simulink library "GPIO_Lib"  (Simulink 8.0)
(part 2 of 2)

      mask TypeOptions Pin7_Speed: GPIO_Speed_2MHz | GPIO_Speed_25MHz | GPIO_Speed_50MHz | GPIO_Speed_100MHz
      mask TypeOptions Pin8_Speed: GPIO_Speed_2MHz | GPIO_Speed_25MHz | GPIO_Speed_50MHz | GPIO_Speed_100MHz
      mask TypeOptions Pin9_Speed: GPIO_Speed_2MHz | GPIO_Speed_25MHz | GPIO_Speed_50MHz | GPIO_Speed_100MHz
      mask TypeOptions Pin10_Speed: GPIO_Speed_2MHz | GPIO_Speed_25MHz | GPIO_Speed_50MHz | GPIO_Speed_100MHz
      mask TypeOptions Pin11_Speed: GPIO_Speed_2MHz | GPIO_Speed_25MHz | GPIO_Speed_50MHz | GPIO_Speed_100MHz
      mask TypeOptions Pin12_Speed: GPIO_Speed_2MHz | GPIO_Speed_25MHz | GPIO_Speed_50MHz | GPIO_Speed_100MHz
      mask TypeOptions Pin13_Speed: GPIO_Speed_2MHz | GPIO_Speed_25MHz | GPIO_Speed_50MHz | GPIO_Speed_100MHz
      mask TypeOptions Pin14_Speed: GPIO_Speed_2MHz | GPIO_Speed_25MHz | GPIO_Speed_50MHz | GPIO_Speed_100MHz
      mask TypeOptions Pin15_Speed: GPIO_Speed_2MHz | GPIO_Speed_25MHz | GPIO_Speed_50MHz | GPIO_Speed_100MHz
      mask TypeOptions Pin0_Mode: GPIO_Mode_IN | GPIO_Mode_OUT | GPIO_Mode_AF | GPIO_Mode_AN
      mask Callback Pin0_Mode: GPIOG_Config_callback('mode0');
      mask TypeOptions Pin1_Mode: GPIO_Mode_IN | GPIO_Mode_OUT | GPIO_Mode_AF | GPIO_Mode_AN
      mask Callback Pin1_Mode: GPIOG_Config_callback('mode1');
      mask TypeOptions Pin2_Mode: GPIO_Mode_IN | GPIO_Mode_OUT | GPIO_Mode_AF | GPIO_Mode_AN
      mask Callback Pin2_Mode: GPIOG_Config_callback('mode2');
      mask TypeOptions Pin3_Mode: GPIO_Mode_IN | GPIO_Mode_OUT | GPIO_Mode_AF | GPIO_Mode_AN
      mask Callback Pin3_Mode: GPIOG_Config_callback('mode3');
      mask TypeOptions Pin4_Mode: GPIO_Mode_IN | GPIO_Mode_OUT | GPIO_Mode_AF | GPIO_Mode_AN
      mask Callback Pin4_Mode: GPIOA_Config_callback('mode4');
      mask TypeOptions Pin5_Mode: GPIO_Mode_IN | GPIO_Mode_OUT | GPIO_Mode_AF | GPIO_Mode_AN
      mask Callback Pin5_Mode: GPIOG_Config_callback('mode5');
      mask TypeOptions Pin6_Mode: GPIO_Mode_IN | GPIO_Mode_OUT | GPIO_Mode_AF | GPIO_Mode_AN
      mask Callback Pin6_Mode: GPIOG_Config_callback('mode6');
      mask TypeOptions Pin7_Mode: GPIO_Mode_IN | GPIO_Mode_OUT | GPIO_Mode_AF | GPIO_Mode_AN
      mask Callback Pin7_Mode: GPIOG_Config_callback('mode7');
      mask TypeOptions Pin8_Mode: GPIO_Mode_IN | GPIO_Mode_OUT | GPIO_Mode_AF | GPIO_Mode_AN
      mask Callback Pin8_Mode: GPIOG_Config_callback('mode8');
      mask TypeOptions Pin9_Mode: GPIO_Mode_IN | GPIO_Mode_OUT | GPIO_Mode_AF | GPIO_Mode_AN
      mask Callback Pin9_Mode: GPIOG_Config_callback('mode9');
      mask TypeOptions Pin10_Mode: GPIO_Mode_IN | GPIO_Mode_OUT | GPIO_Mode_AF | GPIO_Mode_AN
      mask Callback Pin10_Mode: GPIOG_Config_callback('mode10');
      mask TypeOptions Pin11_Mode: GPIO_Mode_IN | GPIO_Mode_OUT | GPIO_Mode_AF | GPIO_Mode_AN
      mask Callback Pin11_Mode: GPIOG_Config_callback('mode11');
      mask TypeOptions Pin12_Mode: GPIO_Mode_IN | GPIO_Mode_OUT | GPIO_Mode_AF | GPIO_Mode_AN
      mask Callback Pin12_Mode: GPIOG_Config_callback('mode12');
      mask TypeOptions Pin13_Mode: GPIO_Mode_IN | GPIO_Mode_OUT | GPIO_Mode_AF | GPIO_Mode_AN
      mask Callback Pin13_Mode: GPIOG_Config_callback('mode13');
      mask TypeOptions Pin14_Mode: GPIO_Mode_IN | GPIO_Mode_OUT | GPIO_Mode_AF | GPIO_Mode_AN
      mask Callback Pin14_Mode: GPIOG_Config_callback('mode14');
      mask TypeOptions Pin15_Mode: GPIO_Mode_IN | GPIO_Mode_OUT | GPIO_Mode_AF | GPIO_Mode_AN
      mask Callback Pin15_Mode: GPIOG_Config_callback('mode15');
      mask TypeOptions Pin0_Type: GPIO_OType_PP | GPIO_OType_OD
      mask TypeOptions Pin1_Type: GPIO_OType_PP | GPIO_OType_OD
      mask TypeOptions Pin2_Type: GPIO_OType_PP | GPIO_OType_OD
      mask TypeOptions Pin3_Type: GPIO_OType_PP | GPIO_OType_OD
      mask TypeOptions Pin4_Type: GPIO_OType_PP | GPIO_OType_OD
      mask TypeOptions Pin5_Type: GPIO_OType_PP | GPIO_OType_OD
      mask TypeOptions Pin6_Type: GPIO_OType_PP | GPIO_OType_OD
      mask TypeOptions Pin7_Type: GPIO_OType_PP | GPIO_OType_OD
      mask TypeOptions Pin8_Type: GPIO_OType_PP | GPIO_OType_OD
      mask TypeOptions Pin9_Type: GPIO_OType_PP | GPIO_OType_OD
      mask TypeOptions Pin10_Type: GPIO_OType_PP | GPIO_OType_OD
      mask TypeOptions Pin11_Type: GPIO_OType_PP | GPIO_OType_OD
      mask TypeOptions Pin12_Type: GPIO_OType_PP | GPIO_OType_OD
      mask TypeOptions Pin13_Type: GPIO_OType_PP | GPIO_OType_OD
      mask TypeOptions Pin14_Type: GPIO_OType_PP | GPIO_OType_OD
      mask TypeOptions Pin15_Type: GPIO_OType_PP | GPIO_OType_OD
      mask TypeOptions Pin0_PuPd: GPIO_PuPd_NOPULL | GPIO_PuPd_UP | GPIO_PuPd_DOWN
      mask TypeOptions Pin1_PuPd: GPIO_PuPd_NOPULL | GPIO_PuPd_UP | GPIO_PuPd_DOWN
      mask TypeOptions Pin2_PuPd: GPIO_PuPd_NOPULL | GPIO_PuPd_UP | GPIO_PuPd_DOWN
      mask TypeOptions Pin3_PuPd: GPIO_PuPd_NOPULL | GPIO_PuPd_UP | GPIO_PuPd_DOWN
      mask TypeOptions Pin4_PuPd: GPIO_PuPd_NOPULL | GPIO_PuPd_UP | GPIO_PuPd_DOWN
      mask TypeOptions Pin5_PuPd: GPIO_PuPd_NOPULL | GPIO_PuPd_UP | GPIO_PuPd_DOWN
      mask TypeOptions Pin6_PuPd: GPIO_PuPd_NOPULL | GPIO_PuPd_UP | GPIO_PuPd_DOWN
      mask TypeOptions Pin7_PuPd: GPIO_PuPd_NOPULL | GPIO_PuPd_UP | GPIO_PuPd_DOWN
      mask TypeOptions Pin8_PuPd: GPIO_PuPd_NOPULL | GPIO_PuPd_UP | GPIO_PuPd_DOWN
      mask TypeOptions Pin9_PuPd: GPIO_PuPd_NOPULL | GPIO_PuPd_UP | GPIO_PuPd_DOWN
      mask TypeOptions Pin10_PuPd: GPIO_PuPd_NOPULL | GPIO_PuPd_UP | GPIO_PuPd_DOWN
      mask TypeOptions Pin11_PuPd: GPIO_PuPd_NOPULL | GPIO_PuPd_UP | GPIO_PuPd_DOWN
      mask TypeOptions Pin12_PuPd: GPIO_PuPd_NOPULL | GPIO_PuPd_UP | GPIO_PuPd_DOWN
      mask TypeOptions Pin13_PuPd: GPIO_PuPd_NOPULL | GPIO_PuPd_UP | GPIO_PuPd_DOWN
      mask TypeOptions Pin14_PuPd: GPIO_PuPd_NOPULL | GPIO_PuPd_UP | GPIO_PuPd_DOWN
      mask TypeOptions Pin15_PuPd: GPIO_PuPd_NOPULL | GPIO_PuPd_UP | GPIO_PuPd_DOWN
      mask TypeOptions Pin0_AF: GPIO_AF_FSMC | GPIO_AF_EVENTOUT
      mask TypeOptions Pin1_AF: GPIO_AF_FSMC | GPIO_AF_EVENTOUT
      mask TypeOptions Pin2_AF: GPIO_AF_FSMC | GPIO_AF_EVENTOUT
      mask TypeOptions Pin3_AF: GPIO_AF_FSMC | GPIO_AF_EVENTOUT
      mask TypeOptions Pin4_AF: GPIO_AF_FSMC | GPIO_AF_EVENTOUT
      mask TypeOptions Pin5_AF: GPIO_AF_FSMC | GPIO_AF_EVENTOUT
      mask TypeOptions Pin6_AF: GPIO_AF_FSMC | GPIO_AF_EVENTOUT
      mask TypeOptions Pin7_AF: GPIO_AF_USART6 | GPIO_AF_FSMC | GPIO_AF_EVENTOUT
      mask TypeOptions Pin8_AF: GPIO_AF_USART6 | GPIO_AF_ETH | GPIO_AF_EVENTOUT
      mask TypeOptions Pin9_AF: GPIO_AF_USART6 | GPIO_AF_FSMC | GPIO_AF_EVENTOUT
      mask TypeOptions Pin10_AF: GPIO_AF_FSMC | GPIO_AF_EVENTOUT
      mask TypeOptions Pin11_AF: GPIO_AF_ETH | GPIO_AF_FSMC | GPIO_AF_EVENTOUT
      mask TypeOptions Pin12_AF: GPIO_AF_USART6 | GPIO_AF_FSMC | GPIO_AF_EVENTOUT
      mask TypeOptions Pin13_AF: GPIO_AF_USART6 | GPIO_AF_ETH | GPIO_AF_FSMC | GPIO_AF_EVENTOUT
      mask TypeOptions Pin14_AF: GPIO_AF_USART6 | GPIO_AF_ETH | GPIO_AF_FSMC | GPIO_AF_EVENTOUT
      mask TypeOptions Pin15_AF: GPIO_AF_USART6 | GPIO_AF_DCMI | GPIO_AF_EVENTOUT
      mask Display:
      | color('blue'); text(0.6, 0.90, 'STM32F4xx', 'horizontalalignment', 'right');color('black'); text(0.50, 0.12, 'GPIOG_Config', 'horizontalAlignment','center');
      | image(imread('ST.bmp','bmp'),'top-right');
  GPIOH_Config : S-Function  LoadFcn=|  FunctionName=GPIOH_Config  Parameters=Pin0_Use,Pin1_Use,Pin2_Use,Pin3_Use,Pin4_Use,Pin5_Use,Pin6_Use,Pin7_Use,Pin8_Use,Pin9_Use,Pin10_Use,Pin11_Use,Pin12_Use,Pin13_Use,Pin14_Use,Pin15_Use,Pin0_Speed,Pin1_Speed,Pin2_Speed,Pin3_Speed,Pin4_Speed,Pin5_Speed,Pin6_Speed,Pin7_Speed,Pin8_Speed,Pin9_Speed,Pin10_Speed,Pin11_Speed,Pin12_Speed,Pin13_Speed,Pin14_Speed,Pin15_Speed,Pin0_Mode,Pin1_Mode,Pin2_Mode,Pin3_Mode,Pin4_Mode,Pin5_Mode,Pin6_Mode,Pin7_Mode,Pin8_Mode,Pin9_Mode,Pin10_Mode,Pin11_Mode,Pin12_Mode,Pin13_Mode,Pin14_Mode,Pin15_Mode,Pin0_Type,Pin1_Type,Pin2_Type,Pin3_Type,Pin4_Type,Pin5_Type,Pin6_Type,Pin7_Type,Pin8_Type,Pin9_Type,Pin10_Type,Pin11_Type,Pin12_Type,Pin13_Type,Pin14_Type,Pin15_Type,Pin0_PuPd,Pin1_PuPd,Pin2_PuPd,Pin3_PuPd,Pin4_PuPd,Pin5_PuPd,Pin6_PuPd,Pin7_PuPd,Pin8_PuPd,Pin9_PuPd,Pin10_PuPd,Pin11_PuPd,Pin12_PuPd,Pin13_PuPd,Pin14_PuPd,Pin15_PuPd,Pin2_AF,Pin3_AF,Pin4_AF,Pin5_AF,Pin6_AF,Pin7_AF,Pin8_AF,Pin9_AF,Pin10_AF,Pin11_AF,Pin12_AF,Pin13_AF,Pin14_AF,Pin15_AF,Pin0_Set,Pin1_Set,Pin2_Set,Pin3_Set,Pin4_Set,Pin5_Set,Pin6_Set,Pin7_Set,Pin8_Set,Pin9_Set,Pin10_Set,Pin11_Set,Pin12_Set,Pin13_Set,Pin14_Set,Pin15_Set  EnableBusSupport=off  mask(GPIOH_Config){Pin0_Use=off, Pin1_Use=off, Pin2_Use=off, Pin3_Use=off, Pin4_Use=off, Pin5_Use=off, Pin6_Use=off, Pin7_Use=off, Pin8_Use=off, Pin9_Use=off, Pin10_Use=off, Pin11_Use=off, Pin12_Use=off, Pin13_Use=off, Pin14_Use=off, Pin15_Use=off, Pin0_Speed=GPIO_Speed_2MHz, Pin1_Speed=GPIO_Speed_2MHz, Pin2_Speed=GPIO_Speed_2MHz, Pin3_Speed=GPIO_Speed_2MHz, Pin4_Speed=GPIO_Speed_2MHz, Pin5_Speed=GPIO_Speed_2MHz, Pin6_Speed=GPIO_Speed_2MHz, Pin7_Speed=GPIO_Speed_2MHz, Pin8_Speed=GPIO_Speed_2MHz, Pin9_Speed=GPIO_Speed_2MHz, Pin10_Speed=GPIO_Speed_2MHz, Pin11_Speed=GPIO_Speed_2MHz, Pin12_Speed=GPIO_Speed_2MHz, Pin13_Speed=GPIO_Speed_2MHz, Pin14_Speed=GPIO_Speed_2MHz, Pin15_Speed=GPIO_Speed_2MHz, Pin0_Mode=GPIO_Mode_OUT, Pin1_Mode=GPIO_Mode_OUT, Pin2_Mode=GPIO_Mode_OUT, Pin3_Mode=GPIO_Mode_OUT, Pin4_Mode=GPIO_Mode_OUT, Pin5_Mode=GPIO_Mode_OUT, Pin6_Mode=GPIO_Mode_OUT, Pin7_Mode=GPIO_Mode_OUT, Pin8_Mode=GPIO_Mode_OUT, Pin9_Mode=GPIO_Mode_OUT, Pin10_Mode=GPIO_Mode_OUT, Pin11_Mode=GPIO_Mode_OUT, Pin12_Mode=GPIO_Mode_OUT, Pin13_Mode=GPIO_Mode_OUT, Pin14_Mode=GPIO_Mode_OUT, Pin15_Mode=GPIO_Mode_OUT, Pin0_Type=GPIO_OType_PP, Pin1_Type=GPIO_OType_PP, Pin2_Type=GPIO_OType_PP, Pin3_Type=GPIO_OType_PP, Pin4_Type=GPIO_OType_PP, Pin5_Type=GPIO_OType_PP, Pin6_Type=GPIO_OType_PP, Pin7_Type=GPIO_OType_PP, Pin8_Type=GPIO_OType_PP, Pin9_Type=GPIO_OType_PP, Pin10_Type=GPIO_OType_PP, Pin11_Type=GPIO_OType_PP, Pin12_Type=GPIO_OType_PP, Pin13_Type=GPIO_OType_PP, Pin14_Type=GPIO_OType_PP, Pin15_Type=GPIO_OType_PP, Pin0_PuPd=GPIO_PuPd_NOPULL, Pin1_PuPd=GPIO_PuPd_NOPULL, Pin2_PuPd=GPIO_PuPd_NOPULL, Pin3_PuPd=GPIO_PuPd_NOPULL, Pin4_PuPd=GPIO_PuPd_NOPULL, Pin5_PuPd=GPIO_PuPd_NOPULL, Pin6_PuPd=GPIO_PuPd_NOPULL, Pin7_PuPd=GPIO_PuPd_NOPULL, Pin8_PuPd=GPIO_PuPd_NOPULL, Pin9_PuPd=GPIO_PuPd_NOPULL, Pin10_PuPd=GPIO_PuPd_NOPULL, Pin11_PuPd=GPIO_PuPd_NOPULL, Pin12_PuPd=GPIO_PuPd_NOPULL, Pin13_PuPd=GPIO_PuPd_NOPULL, Pin14_PuPd=GPIO_PuPd_NOPULL, Pin15_PuPd=GPIO_PuPd_NOPULL, Pin2_AF=GPIO_AF_ETH, Pin3_AF=GPIO_AF_ETH, Pin4_AF=GPIO_AF_I2C2, Pin5_AF=GPIO_AF_EVENTOUT, Pin6_AF=GPIO_AF_I2C2, Pin7_AF=GPIO_AF_I2C3, Pin8_AF=GPIO_AF_I2C3, Pin9_AF=GPIO_AF_I2C3, Pin10_AF=GPIO_AF_TIM5, Pin11_AF=GPIO_AF_TIM5, Pin12_AF=GPIO_AF_TIM5, Pin13_AF=GPIO_AF_TIM8, Pin14_AF=GPIO_AF_TIM8, Pin15_AF=GPIO_AF_EVENTOUT, Pin0_Set=off, Pin1_Set=off, Pin2_Set=off, Pin3_Set=off, Pin4_Set=off, Pin5_Set=off, Pin6_Set=off, Pin7_Set=off, Pin8_Set=off, Pin9_Set=off, Pin10_Set=off, Pin11_Set=off, Pin12_Set=off, Pin13_Set=off, Pin14_Set=off, Pin15_Set=off}
      | libFiles =    updatePrefs('get','stm32f4listLibFiles');          libFiles2Build = updatePrefs('get','stm32f4listLibBuildFiles');
      |                                                                                                                                 
      | gpio = strcmp('stm32f4xx_gpio.c',{libFiles(:).name});                                                                           
      | libFiles2Build(gpio) = libFiles2Build(gpio) + 1;                                                                                
      | rcc = strcmp('stm32f4xx_rcc.c',{libFiles(:).name}) ;                                                                            
      | libFiles2Build(rcc) = libFiles2Build(rcc) + 1;                                                                                  
      |                                                                                                                                 
      | updatePrefs('set','stm32f4listLibBuildFiles',libFiles2Build);                                                                   
      | clear gpio rcc  libFiles                                                                                                        
      | clear libFiles2Build
      mask prompts: Pin0_Use "Pin used"; Pin1_Use "Pin used"; Pin2_Use "Pin used"; Pin3_Use "Pin used"; Pin4_Use "Pin used"; Pin5_Use "Pin used"; Pin6_Use "Pin used"; Pin7_Use "Pin used"; Pin8_Use "Pin used"; Pin9_Use "Pin used"; Pin10_Use "Pin used"; Pin11_Use "Pin used"; Pin12_Use "Pin used"; Pin13_Use "Pin used"; Pin14_Use "Pin used"; Pin15_Use "Pin used"; Pin0_Speed "Maximum frequency"; Pin1_Speed "Maximum frequency"; Pin2_Speed "Maximum frequency"; Pin3_Speed "Maximum frequency"; Pin4_Speed "Maximum frequency"; Pin5_Speed "Maximum frequency"; Pin6_Speed "Maximum frequency"; Pin7_Speed "Maximum frequency"; Pin8_Speed "Maximum frequency"; Pin9_Speed "Maximum frequency"; Pin10_Speed "Maximum frequency"; Pin11_Speed "Maximum frequency"; Pin12_Speed "Maximum frequency"; Pin13_Speed "Maximum frequency"; Pin14_Speed "Maximum frequency"; Pin15_Speed "Maximum frequency"; Pin0_Mode "Configuration mode"; Pin1_Mode "Configuration mode"; Pin2_Mode "Configuration mode"; Pin3_Mode "Configuration mode"; Pin4_Mode "Configuration mode"; Pin5_Mode "Configuration mode"; Pin6_Mode "Configuration mode"; Pin7_Mode "Configuration mode"; Pin8_Mode "Configuration mode"; Pin9_Mode "Configuration mode"; Pin10_Mode "Configuration mode"; Pin11_Mode "Configuration mode"; Pin12_Mode "Configuration mode"; Pin13_Mode "Configuration mode"; Pin14_Mode "Configuration mode"; Pin15_Mode "Configuration mode"; Pin0_Type "Configuration output type"; Pin1_Type "Configuration output type"; Pin2_Type "Configuration output type"; Pin3_Type "Configuration output type"; Pin4_Type "Configuration output type"; Pin5_Type "Configuration output type"; Pin6_Type "Configuration output type"; Pin7_Type "Configuration output type"; Pin8_Type "Configuration output type"; Pin9_Type "Configuration output type"; Pin10_Type "Configuration output type"; Pin11_Type "Configuration output type"; Pin12_Type "Configuration output type"; Pin13_Type "Configuration output type"; Pin14_Type "Configuration output type"; Pin15_Type "Configuration output type"; Pin0_PuPd "Configuration PullUp PullDown"; Pin1_PuPd "Configuration PullUp PullDown"; Pin2_PuPd "Configuration PullUp PullDown"; Pin3_PuPd "Configuration PullUp PullDown"; Pin4_PuPd "Configuration PullUp PullDown"; Pin5_PuPd "Configuration PullUp PullDown"; Pin6_PuPd "Configuration PullUp PullDown"; Pin7_PuPd "Configuration PullUp PullDown"; Pin8_PuPd "Configuration PullUp PullDown"; Pin9_PuPd "Configuration PullUp PullDown"; Pin10_PuPd "Configuration PullUp PullDown"; Pin11_PuPd "Configuration PullUp PullDown"; Pin12_PuPd "Configuration PullUp PullDown"; Pin13_PuPd "Configuration PullUp PullDown"; Pin14_PuPd "Configuration PullUp PullDown"; Pin15_PuPd "Configuration PullUp PullDown"; Pin2_AF "Alternate Function"; Pin3_AF "Alternate Function"; Pin4_AF "Alternate Function"; Pin5_AF "Alternate Function"; Pin6_AF "Alternate Function"; Pin7_AF "Alternate Function"; Pin8_AF "Alternate Function"; Pin9_AF "Alternate Function"; Pin10_AF "Alternate Function"; Pin11_AF "Alternate Function"; Pin12_AF "Alternate Function"; Pin13_AF "Alternate Function"; Pin14_AF "Alternate Function"; Pin15_AF "Alternate Function"; Pin0_Set "Set High initial value"; Pin1_Set "Set High initial value"; Pin2_Set "Set High initial value"; Pin3_Set "Set High initial value"; Pin4_Set "Set High initial value"; Pin5_Set "Set High initial value"; Pin6_Set "Set High initial value"; Pin7_Set "Set High initial value"; Pin8_Set "Set High initial value"; Pin9_Set "Set High initial value"; Pin10_Set "Set High initial value"; Pin11_Set "Set High initial value"; Pin12_Set "Set High initial value"; Pin13_Set "Set High initial value"; Pin14_Set "Set High initial value"; Pin15_Set "Set High initial value"
      mask help:
      | GPIO (General Purpose In/Out) PortH configuration:
      | Configure PortH, Pin0 to Pin15 as input, output, Analogic or Alternate function.
      | Maximum GPIO speed is 2Mhz, 25Mhz, 50Mhz or 100Mhz.
      | Output is PushPull or OpenDrain.
      | Input is PullUp, PullDown, PullUpPullDown or No pull.
      | Alternate function is different for each pin. (No AF for Pin0 and Pin1)
      settings: CopyFcn=|
      | pathTmf = updatePrefs('get','stm32f4RootPath');
      | if isempty(pathTmf)
      | h = errordlg('Add STM32F4xx repository to Matlab default path or set System target file to stm32F4xx.tlc before!' ,'STM32F4xx','modal');
      | close(h);
      | clear h
      | end
      | libFiles =    updatePrefs('get','stm32f4listLibFiles');          libFiles2Build = updatePrefs('get','stm32f4listLibBuildFiles');
      | gpio = strcmp('stm32f4xx_gpio.c',{libFiles(:).name});
      | libFiles2Build(gpio) = libFiles2Build(gpio) + 1;
      | rcc = strcmp('stm32f4xx_rcc.c',{libFiles(:).name}) ;
      | libFiles2Build(rcc) = libFiles2Build(rcc) + 1;
      | updatePrefs('set','stm32f4listLibBuildFiles',libFiles2Build);
      | clear gpio rcc  pathTmf libFiles
      | clear libFiles2Build
      settings: DeleteFcn=|
      | libFiles =    updatePrefs('get','stm32f4listLibFiles');          libFiles2Build = updatePrefs('get','stm32f4listLibBuildFiles');
      | gpio = strcmp('stm32f4xx_gpio.c',{libFiles(:).name});
      | libFiles2Build(gpio) = libFiles2Build(gpio) - 1;  if(libFiles2Build(gpio) <0)
      | libFiles2Build(gpio)  = 0;                                  end
      | rcc = strcmp('stm32f4xx_rcc.c',{libFiles(:).name}) ;
      | libFiles2Build(rcc) = libFiles2Build(rcc) - 1;    if(libFiles2Build(rcc) <0)
      | libFiles2Build(rcc)  = 0;                                  end
      | updatePrefs('set','stm32f4listLibBuildFiles',libFiles2Build);
      | clear gpio rcc  libFiles  libFiles2Build
      settings: UndoDeleteFcn=|
      | libFiles =    updatePrefs('get','stm32f4listLibFiles');          libFiles2Build = updatePrefs('get','stm32f4listLibBuildFiles');
      | gpio = strcmp('stm32f4xx_gpio.c',{libFiles(:).name});
      | libFiles2Build(gpio) = libFiles2Build(gpio) + 1;
      | rcc = strcmp('stm32f4xx_rcc.c',{libFiles(:).name}) ;
      | libFiles2Build(rcc) = libFiles2Build(rcc) + 1;
      | updatePrefs('set','stm32f4listLibBuildFiles',libFiles2Build);
      | clear gpio rcc  libFiles
      | clear libFiles2Build
      mask Help: web('help_GPIOH_Config.html', '-helpbrowser')
      mask Callback Pin0_Use: GPIOH_Config_callback('use0');
      mask Callback Pin1_Use: GPIOH_Config_callback('use1');
      mask Callback Pin2_Use: GPIOH_Config_callback('use2');
      mask Callback Pin3_Use: GPIOH_Config_callback('use3');
      mask Callback Pin4_Use: GPIOH_Config_callback('use4');
      mask Callback Pin5_Use: GPIOH_Config_callback('use5');
      mask Callback Pin6_Use: GPIOH_Config_callback('use6');
      mask Callback Pin7_Use: GPIOH_Config_callback('use7');
      mask Callback Pin8_Use: GPIOH_Config_callback('use8');
      mask Callback Pin9_Use: GPIOH_Config_callback('use9');
      mask Callback Pin10_Use: GPIOA_Config_callback('use10');
      mask Callback Pin11_Use: GPIOH_Config_callback('use11');
      mask Callback Pin12_Use: GPIOH_Config_callback('use12');
      mask Callback Pin13_Use: GPIOH_Config_callback('use13');
      mask Callback Pin14_Use: GPIOH_Config_callback('use14');
      mask Callback Pin15_Use: GPIOH_Config_callback('use15');
      mask TypeOptions Pin0_Speed: GPIO_Speed_2MHz | GPIO_Speed_25MHz | GPIO_Speed_50MHz | GPIO_Speed_100MHz
      mask TypeOptions Pin1_Speed: GPIO_Speed_2MHz | GPIO_Speed_25MHz | GPIO_Speed_50MHz | GPIO_Speed_100MHz
      mask TypeOptions Pin2_Speed: GPIO_Speed_2MHz | GPIO_Speed_25MHz | GPIO_Speed_50MHz | GPIO_Speed_100MHz
      mask TypeOptions Pin3_Speed: GPIO_Speed_2MHz | GPIO_Speed_25MHz | GPIO_Speed_50MHz | GPIO_Speed_100MHz
      mask TypeOptions Pin4_Speed: GPIO_Speed_2MHz | GPIO_Speed_25MHz | GPIO_Speed_50MHz | GPIO_Speed_100MHz
      mask TypeOptions Pin5_Speed: GPIO_Speed_2MHz | GPIO_Speed_25MHz | GPIO_Speed_50MHz | GPIO_Speed_100MHz
      mask TypeOptions Pin6_Speed: GPIO_Speed_2MHz | GPIO_Speed_25MHz | GPIO_Speed_50MHz | GPIO_Speed_100MHz
      mask TypeOptions Pin7_Speed: GPIO_Speed_2MHz | GPIO_Speed_25MHz | GPIO_Speed_50MHz | GPIO_Speed_100MHz
      mask TypeOptions Pin8_Speed: GPIO_Speed_2MHz | GPIO_Speed_25MHz | GPIO_Speed_50MHz | GPIO_Speed_100MHz
      mask TypeOptions Pin9_Speed: GPIO_Speed_2MHz | GPIO_Speed_25MHz | GPIO_Speed_50MHz | GPIO_Speed_100MHz
      mask TypeOptions Pin10_Speed: GPIO_Speed_2MHz | GPIO_Speed_25MHz | GPIO_Speed_50MHz | GPIO_Speed_100MHz
      mask TypeOptions Pin11_Speed: GPIO_Speed_2MHz | GPIO_Speed_25MHz | GPIO_Speed_50MHz | GPIO_Speed_100MHz
      mask TypeOptions Pin12_Speed: GPIO_Speed_2MHz | GPIO_Speed_25MHz | GPIO_Speed_50MHz | GPIO_Speed_100MHz
      mask TypeOptions Pin13_Speed: GPIO_Speed_2MHz | GPIO_Speed_25MHz | GPIO_Speed_50MHz | GPIO_Speed_100MHz
      mask TypeOptions Pin14_Speed: GPIO_Speed_2MHz | GPIO_Speed_25MHz | GPIO_Speed_50MHz | GPIO_Speed_100MHz
      mask TypeOptions Pin15_Speed: GPIO_Speed_2MHz | GPIO_Speed_25MHz | GPIO_Speed_50MHz | GPIO_Speed_100MHz
      mask TypeOptions Pin0_Mode: GPIO_Mode_IN | GPIO_Mode_OUT | GPIO_Mode_AN
      mask Callback Pin0_Mode: GPIOH_Config_callback('mode0');
      mask TypeOptions Pin1_Mode: GPIO_Mode_IN | GPIO_Mode_OUT | GPIO_Mode_AN
      mask Callback Pin1_Mode: GPIOH_Config_callback('mode1');
      mask TypeOptions Pin2_Mode: GPIO_Mode_IN | GPIO_Mode_OUT | GPIO_Mode_AF | GPIO_Mode_AN
      mask Callback Pin2_Mode: GPIOH_Config_callback('mode2');
      mask TypeOptions Pin3_Mode: GPIO_Mode_IN | GPIO_Mode_OUT | GPIO_Mode_AF | GPIO_Mode_AN
      mask Callback Pin3_Mode: GPIOH_Config_callback('mode3');
      mask TypeOptions Pin4_Mode: GPIO_Mode_IN | GPIO_Mode_OUT | GPIO_Mode_AF | GPIO_Mode_AN
      mask Callback Pin4_Mode: GPIOA_Config_callback('mode4');
      mask TypeOptions Pin5_Mode: GPIO_Mode_IN | GPIO_Mode_OUT | GPIO_Mode_AF | GPIO_Mode_AN
      mask Callback Pin5_Mode: GPIOH_Config_callback('mode5');
      mask TypeOptions Pin6_Mode: GPIO_Mode_IN | GPIO_Mode_OUT | GPIO_Mode_AF | GPIO_Mode_AN
      mask Callback Pin6_Mode: GPIOH_Config_callback('mode6');
      mask TypeOptions Pin7_Mode: GPIO_Mode_IN | GPIO_Mode_OUT | GPIO_Mode_AF | GPIO_Mode_AN
      mask Callback Pin7_Mode: GPIOH_Config_callback('mode7');
      mask TypeOptions Pin8_Mode: GPIO_Mode_IN | GPIO_Mode_OUT | GPIO_Mode_AF | GPIO_Mode_AN
      mask Callback Pin8_Mode: GPIOH_Config_callback('mode8');
      mask TypeOptions Pin9_Mode: GPIO_Mode_IN | GPIO_Mode_OUT | GPIO_Mode_AF | GPIO_Mode_AN
      mask Callback Pin9_Mode: GPIOH_Config_callback('mode9');
      mask TypeOptions Pin10_Mode: GPIO_Mode_IN | GPIO_Mode_OUT | GPIO_Mode_AF | GPIO_Mode_AN
      mask Callback Pin10_Mode: GPIOH_Config_callback('mode10');
      mask TypeOptions Pin11_Mode: GPIO_Mode_IN | GPIO_Mode_OUT | GPIO_Mode_AF | GPIO_Mode_AN
      mask Callback Pin11_Mode: GPIOH_Config_callback('mode11');
      mask TypeOptions Pin12_Mode: GPIO_Mode_IN | GPIO_Mode_OUT | GPIO_Mode_AF | GPIO_Mode_AN
      mask Callback Pin12_Mode: GPIOH_Config_callback('mode12');
      mask TypeOptions Pin13_Mode: GPIO_Mode_IN | GPIO_Mode_OUT | GPIO_Mode_AF | GPIO_Mode_AN
      mask Callback Pin13_Mode: GPIOH_Config_callback('mode13');
      mask TypeOptions Pin14_Mode: GPIO_Mode_IN | GPIO_Mode_OUT | GPIO_Mode_AF | GPIO_Mode_AN
      mask Callback Pin14_Mode: GPIOH_Config_callback('mode14');
      mask TypeOptions Pin15_Mode: GPIO_Mode_IN | GPIO_Mode_OUT | GPIO_Mode_AF | GPIO_Mode_AN
      mask Callback Pin15_Mode: GPIOH_Config_callback('mode15');
      mask TypeOptions Pin0_Type: GPIO_OType_PP | GPIO_OType_OD
      mask TypeOptions Pin1_Type: GPIO_OType_PP | GPIO_OType_OD
      mask TypeOptions Pin2_Type: GPIO_OType_PP | GPIO_OType_OD
      mask TypeOptions Pin3_Type: GPIO_OType_PP | GPIO_OType_OD
      mask TypeOptions Pin4_Type: GPIO_OType_PP | GPIO_OType_OD
      mask TypeOptions Pin5_Type: GPIO_OType_PP | GPIO_OType_OD
      mask TypeOptions Pin6_Type: GPIO_OType_PP | GPIO_OType_OD
      mask TypeOptions Pin7_Type: GPIO_OType_PP | GPIO_OType_OD
      mask TypeOptions Pin8_Type: GPIO_OType_PP | GPIO_OType_OD
      mask TypeOptions Pin9_Type: GPIO_OType_PP | GPIO_OType_OD
      mask TypeOptions Pin10_Type: GPIO_OType_PP | GPIO_OType_OD
      mask TypeOptions Pin11_Type: GPIO_OType_PP | GPIO_OType_OD
      mask TypeOptions Pin12_Type: GPIO_OType_PP | GPIO_OType_OD
      mask TypeOptions Pin13_Type: GPIO_OType_PP | GPIO_OType_OD
      mask TypeOptions Pin14_Type: GPIO_OType_PP | GPIO_OType_OD
      mask TypeOptions Pin15_Type: GPIO_OType_PP | GPIO_OType_OD
      mask TypeOptions Pin0_PuPd: GPIO_PuPd_NOPULL | GPIO_PuPd_UP | GPIO_PuPd_DOWN
      mask TypeOptions Pin1_PuPd: GPIO_PuPd_NOPULL | GPIO_PuPd_UP | GPIO_PuPd_DOWN
      mask TypeOptions Pin2_PuPd: GPIO_PuPd_NOPULL | GPIO_PuPd_UP | GPIO_PuPd_DOWN
      mask TypeOptions Pin3_PuPd: GPIO_PuPd_NOPULL | GPIO_PuPd_UP | GPIO_PuPd_DOWN
      mask TypeOptions Pin4_PuPd: GPIO_PuPd_NOPULL | GPIO_PuPd_UP | GPIO_PuPd_DOWN
      mask TypeOptions Pin5_PuPd: GPIO_PuPd_NOPULL | GPIO_PuPd_UP | GPIO_PuPd_DOWN
      mask TypeOptions Pin6_PuPd: GPIO_PuPd_NOPULL | GPIO_PuPd_UP | GPIO_PuPd_DOWN
      mask TypeOptions Pin7_PuPd: GPIO_PuPd_NOPULL | GPIO_PuPd_UP | GPIO_PuPd_DOWN
      mask TypeOptions Pin8_PuPd: GPIO_PuPd_NOPULL | GPIO_PuPd_UP | GPIO_PuPd_DOWN
      mask TypeOptions Pin9_PuPd: GPIO_PuPd_NOPULL | GPIO_PuPd_UP | GPIO_PuPd_DOWN
      mask TypeOptions Pin10_PuPd: GPIO_PuPd_NOPULL | GPIO_PuPd_UP | GPIO_PuPd_DOWN
      mask TypeOptions Pin11_PuPd: GPIO_PuPd_NOPULL | GPIO_PuPd_UP | GPIO_PuPd_DOWN
      mask TypeOptions Pin12_PuPd: GPIO_PuPd_NOPULL | GPIO_PuPd_UP | GPIO_PuPd_DOWN
      mask TypeOptions Pin13_PuPd: GPIO_PuPd_NOPULL | GPIO_PuPd_UP | GPIO_PuPd_DOWN
      mask TypeOptions Pin14_PuPd: GPIO_PuPd_NOPULL | GPIO_PuPd_UP | GPIO_PuPd_DOWN
      mask TypeOptions Pin15_PuPd: GPIO_PuPd_NOPULL | GPIO_PuPd_UP | GPIO_PuPd_DOWN
      mask TypeOptions Pin2_AF: GPIO_AF_ETH | GPIO_AF_EVENTOUT
      mask TypeOptions Pin3_AF: GPIO_AF_ETH | GPIO_AF_EVENTOUT
      mask TypeOptions Pin4_AF: GPIO_AF_I2C2 | GPIO_AF_OTG_HS | GPIO_AF_EVENTOUT
      mask TypeOptions Pin5_AF: GPIO_AF_I2C2 | GPIO_AF_EVENTOUT
      mask TypeOptions Pin6_AF: GPIO_AF_I2C2 | GPIO_AF_TIM12 | GPIO_AF_ETH | GPIO_AF_EVENTOUT
      mask TypeOptions Pin7_AF: GPIO_AF_I2C3 | GPIO_AF_ETH | GPIO_AF_EVENTOUT
      mask TypeOptions Pin8_AF: GPIO_AF_I2C3 | GPIO_AF_DCMI | GPIO_AF_EVENTOUT
      mask TypeOptions Pin9_AF: GPIO_AF_I2C3 | GPIO_AF_TIM12 | GPIO_AF_DCMI | GPIO_AF_EVENTOUT
      mask TypeOptions Pin10_AF: GPIO_AF_TIM5 | GPIO_AF_DCMI | GPIO_AF_EVENTOUT
      mask TypeOptions Pin11_AF: GPIO_AF_TIM5 | GPIO_AF_DCMI | GPIO_AF_EVENTOUT
      mask TypeOptions Pin12_AF: GPIO_AF_TIM5 | GPIO_AF_DCMI | GPIO_AF_EVENTOUT
      mask TypeOptions Pin13_AF: GPIO_AF_TIM8 | GPIO_AF_CAN1 | GPIO_AF_EVENTOUT
      mask TypeOptions Pin14_AF: GPIO_AF_TIM8 | GPIO_AF_DCMI | GPIO_AF_EVENTOUT
      mask TypeOptions Pin15_AF: GPIO_AF_TIM8 | GPIO_AF_DCMI | GPIO_AF_EVENTOUT
      mask Display:
      | color('blue'); text(0.6, 0.90, 'STM32F4xx', 'horizontalalignment', 'right');color('black'); text(0.50, 0.12, 'GPIOH_Config', 'horizontalAlignment','center');
      | image(imread('ST.bmp','bmp'),'top-right');
  GPIOI_Config : S-Function  LoadFcn=|  FunctionName=GPIOI_Config  Parameters=Pin0_Use,Pin1_Use,Pin2_Use,Pin3_Use,Pin4_Use,Pin5_Use,Pin6_Use,Pin7_Use,Pin8_Use,Pin9_Use,Pin10_Use,Pin11_Use,Pin0_Speed,Pin1_Speed,Pin2_Speed,Pin3_Speed,Pin4_Speed,Pin5_Speed,Pin6_Speed,Pin7_Speed,Pin8_Speed,Pin9_Speed,Pin10_Speed,Pin11_Speed,Pin0_Mode,Pin1_Mode,Pin2_Mode,Pin3_Mode,Pin4_Mode,Pin5_Mode,Pin6_Mode,Pin7_Mode,Pin8_Mode,Pin9_Mode,Pin10_Mode,Pin11_Mode,Pin0_Type,Pin1_Type,Pin2_Type,Pin3_Type,Pin4_Type,Pin5_Type,Pin6_Type,Pin7_Type,Pin8_Type,Pin9_Type,Pin10_Type,Pin11_Type,Pin0_PuPd,Pin1_PuPd,Pin2_PuPd,Pin3_PuPd,Pin4_PuPd,Pin5_PuPd,Pin6_PuPd,Pin7_PuPd,Pin8_PuPd,Pin9_PuPd,Pin10_PuPd,Pin11_PuPd,Pin0_AF,Pin1_AF,Pin2_AF,Pin3_AF,Pin4_AF,Pin5_AF,Pin6_AF,Pin7_AF,Pin9_AF,Pin10_AF,Pin11_AF,Pin0_Set,Pin1_Set,Pin2_Set,Pin3_Set,Pin4_Set,Pin5_Set,Pin6_Set,Pin7_Set,Pin8_Set,Pin9_Set,Pin10_Set,Pin11_Set  EnableBusSupport=off  mask(GPIOI_Config){Pin0_Use=off, Pin1_Use=off, Pin2_Use=off, Pin3_Use=off, Pin4_Use=off, Pin5_Use=off, Pin6_Use=off, Pin7_Use=off, Pin8_Use=off, Pin9_Use=off, Pin10_Use=off, Pin11_Use=off, Pin0_Speed=GPIO_Speed_2MHz, Pin1_Speed=GPIO_Speed_2MHz, Pin2_Speed=GPIO_Speed_2MHz, Pin3_Speed=GPIO_Speed_2MHz, Pin4_Speed=GPIO_Speed_2MHz, Pin5_Speed=GPIO_Speed_2MHz, Pin6_Speed=GPIO_Speed_2MHz, Pin7_Speed=GPIO_Speed_2MHz, Pin8_Speed=GPIO_Speed_2MHz, Pin9_Speed=GPIO_Speed_2MHz, Pin10_Speed=GPIO_Speed_2MHz, Pin11_Speed=GPIO_Speed_2MHz, Pin0_Mode=GPIO_Mode_OUT, Pin1_Mode=GPIO_Mode_OUT, Pin2_Mode=GPIO_Mode_OUT, Pin3_Mode=GPIO_Mode_OUT, Pin4_Mode=GPIO_Mode_OUT, Pin5_Mode=GPIO_Mode_OUT, Pin6_Mode=GPIO_Mode_OUT, Pin7_Mode=GPIO_Mode_OUT, Pin8_Mode=GPIO_Mode_OUT, Pin9_Mode=GPIO_Mode_OUT, Pin10_Mode=GPIO_Mode_OUT, Pin11_Mode=GPIO_Mode_OUT, Pin0_Type=GPIO_OType_PP, Pin1_Type=GPIO_OType_PP, Pin2_Type=GPIO_OType_PP, Pin3_Type=GPIO_OType_PP, Pin4_Type=GPIO_OType_PP, Pin5_Type=GPIO_OType_PP, Pin6_Type=GPIO_OType_PP, Pin7_Type=GPIO_OType_PP, Pin8_Type=GPIO_OType_PP, Pin9_Type=GPIO_OType_PP, Pin10_Type=GPIO_OType_PP, Pin11_Type=GPIO_OType_PP, Pin0_PuPd=GPIO_PuPd_NOPULL, Pin1_PuPd=GPIO_PuPd_NOPULL, Pin2_PuPd=GPIO_PuPd_NOPULL, Pin3_PuPd=GPIO_PuPd_NOPULL, Pin4_PuPd=GPIO_PuPd_NOPULL, Pin5_PuPd=GPIO_PuPd_NOPULL, Pin6_PuPd=GPIO_PuPd_NOPULL, Pin7_PuPd=GPIO_PuPd_NOPULL, Pin8_PuPd=GPIO_PuPd_NOPULL, Pin9_PuPd=GPIO_PuPd_NOPULL, Pin10_PuPd=GPIO_PuPd_NOPULL, Pin11_PuPd=GPIO_PuPd_NOPULL, Pin0_AF=GPIO_AF_TIM5, Pin1_AF=GPIO_AF_SPI2, Pin2_AF=GPIO_AF_TIM8, Pin3_AF=GPIO_AF_TIM8, Pin4_AF=GPIO_AF_TIM8, Pin5_AF=GPIO_AF_EVENTOUT, Pin6_AF=GPIO_AF_TIM8, Pin7_AF=GPIO_AF_TIM8, Pin9_AF=GPIO_AF_CAN1, Pin10_AF=GPIO_AF_ETH, Pin11_AF=GPIO_AF_OTG_HS, Pin0_Set=off, Pin1_Set=off, Pin2_Set=off, Pin3_Set=off, Pin4_Set=off, Pin5_Set=off, Pin6_Set=off, Pin7_Set=off, Pin8_Set=off, Pin9_Set=off, Pin10_Set=off, Pin11_Set=off}
      | libFiles =    updatePrefs('get','stm32f4listLibFiles');          libFiles2Build = updatePrefs('get','stm32f4listLibBuildFiles');
      |                                                                                                                                 
      | gpio = strcmp('stm32f4xx_gpio.c',{libFiles(:).name});                                                                           
      | libFiles2Build(gpio) = libFiles2Build(gpio) + 1;                                                                                
      | rcc = strcmp('stm32f4xx_rcc.c',{libFiles(:).name}) ;                                                                            
      | libFiles2Build(rcc) = libFiles2Build(rcc) + 1;                                                                                  
      |                                                                                                                                 
      | updatePrefs('set','stm32f4listLibBuildFiles',libFiles2Build);                                                                   
      | clear gpio rcc  libFiles                                                                                                        
      | clear libFiles2Build
      mask prompts: Pin0_Use "Pin used"; Pin1_Use "Pin used"; Pin2_Use "Pin used"; Pin3_Use "Pin used"; Pin4_Use "Pin used"; Pin5_Use "Pin used"; Pin6_Use "Pin used"; Pin7_Use "Pin used"; Pin8_Use "Pin used"; Pin9_Use "Pin used"; Pin10_Use "Pin used"; Pin11_Use "Pin used"; Pin0_Speed "Maximum frequency"; Pin1_Speed "Maximum frequency"; Pin2_Speed "Maximum frequency"; Pin3_Speed "Maximum frequency"; Pin4_Speed "Maximum frequency"; Pin5_Speed "Maximum frequency"; Pin6_Speed "Maximum frequency"; Pin7_Speed "Maximum frequency"; Pin8_Speed "Maximum frequency"; Pin9_Speed "Maximum frequency"; Pin10_Speed "Maximum frequency"; Pin11_Speed "Maximum frequency"; Pin0_Mode "Configuration mode"; Pin1_Mode "Configuration mode"; Pin2_Mode "Configuration mode"; Pin3_Mode "Configuration mode"; Pin4_Mode "Configuration mode"; Pin5_Mode "Configuration mode"; Pin6_Mode "Configuration mode"; Pin7_Mode "Configuration mode"; Pin8_Mode "Configuration mode"; Pin9_Mode "Configuration mode"; Pin10_Mode "Configuration mode"; Pin11_Mode "Configuration mode"; Pin0_Type "Configuration output type"; Pin1_Type "Configuration output type"; Pin2_Type "Configuration output type"; Pin3_Type "Configuration output type"; Pin4_Type "Configuration output type"; Pin5_Type "Configuration output type"; Pin6_Type "Configuration output type"; Pin7_Type "Configuration output type"; Pin8_Type "Configuration output type"; Pin9_Type "Configuration output type"; Pin10_Type "Configuration output type"; Pin11_Type "Configuration output type"; Pin0_PuPd "Configuration PullUp PullDown"; Pin1_PuPd "Configuration PullUp PullDown"; Pin2_PuPd "Configuration PullUp PullDown"; Pin3_PuPd "Configuration PullUp PullDown"; Pin4_PuPd "Configuration PullUp PullDown"; Pin5_PuPd "Configuration PullUp PullDown"; Pin6_PuPd "Configuration PullUp PullDown"; Pin7_PuPd "Configuration PullUp PullDown"; Pin8_PuPd "Configuration PullUp PullDown"; Pin9_PuPd "Configuration PullUp PullDown"; Pin10_PuPd "Configuration PullUp PullDown"; Pin11_PuPd "Configuration PullUp PullDown"; Pin0_AF "Alternate Function"; Pin1_AF "Alternate Function"; Pin2_AF "Alternate Function"; Pin3_AF "Alternate Function"; Pin4_AF "Alternate Function"; Pin5_AF "Alternate Function"; Pin6_AF "Alternate Function"; Pin7_AF "Alternate Function"; Pin9_AF "Alternate Function"; Pin10_AF "Alternate Function"; Pin11_AF "Alternate Function"; Pin0_Set "Set High initial value"; Pin1_Set "Set High initial value"; Pin2_Set "Set High initial value"; Pin3_Set "Set High initial value"; Pin4_Set "Set High initial value"; Pin5_Set "Set High initial value"; Pin6_Set "Set High initial value"; Pin7_Set "Set High initial value"; Pin8_Set "Set High initial value"; Pin9_Set "Set High initial value"; Pin10_Set "Set High initial value"; Pin11_Set "Set High initial value"
      mask help:
      | GPIO (General Purpose In/Out) PortI configuration:
      | Configure PortI, Pin0 to Pin11 as input, output, Analogic or Alternate function.
      | Maximum GPIO speed is 2Mhz, 25Mhz, 50Mhz or 100Mhz.
      | Output is PushPull or OpenDrain.
      | Input is PullUp, PullDown, PullUpPullDown or No pull.
      | Alternate function is different for each pin (No AF for pin8)
      settings: CopyFcn=|
      | pathTmf = updatePrefs('get','stm32f4RootPath');
      | if isempty(pathTmf)
      | h = errordlg('Add STM32F4xx repository to Matlab default path or set System target file to stm32F4xx.tlc before!' ,'STM32F4xx','modal');
      | close(h);
      | clear h
      | end
      | libFiles =    updatePrefs('get','stm32f4listLibFiles');          libFiles2Build = updatePrefs('get','stm32f4listLibBuildFiles');
      | gpio = strcmp('stm32f4xx_gpio.c',{libFiles(:).name});
      | libFiles2Build(gpio) = libFiles2Build(gpio) + 1;
      | rcc = strcmp('stm32f4xx_rcc.c',{libFiles(:).name}) ;
      | libFiles2Build(rcc) = libFiles2Build(rcc) + 1;
      | updatePrefs('set','stm32f4listLibBuildFiles',libFiles2Build);
      | clear gpio rcc  pathTmf libFiles
      | clear libFiles2Build
      settings: DeleteFcn=|
      | libFiles =    updatePrefs('get','stm32f4listLibFiles');          libFiles2Build = updatePrefs('get','stm32f4listLibBuildFiles');
      | gpio = strcmp('stm32f4xx_gpio.c',{libFiles(:).name});
      | libFiles2Build(gpio) = libFiles2Build(gpio) - 1;  if(libFiles2Build(gpio) <0)
      | libFiles2Build(gpio)  = 0;                                  end
      | rcc = strcmp('stm32f4xx_rcc.c',{libFiles(:).name}) ;
      | libFiles2Build(rcc) = libFiles2Build(rcc) - 1;    if(libFiles2Build(rcc) <0)
      | libFiles2Build(rcc)  = 0;                                  end
      | updatePrefs('set','stm32f4listLibBuildFiles',libFiles2Build);
      | clear gpio rcc  libFiles  libFiles2Build
      settings: UndoDeleteFcn=|
      | libFiles =    updatePrefs('get','stm32f4listLibFiles');          libFiles2Build = updatePrefs('get','stm32f4listLibBuildFiles');
      | gpio = strcmp('stm32f4xx_gpio.c',{libFiles(:).name});
      | libFiles2Build(gpio) = libFiles2Build(gpio) + 1;
      | rcc = strcmp('stm32f4xx_rcc.c',{libFiles(:).name}) ;
      | libFiles2Build(rcc) = libFiles2Build(rcc) + 1;
      | updatePrefs('set','stm32f4listLibBuildFiles',libFiles2Build);
      | clear gpio rcc  libFiles
      | clear libFiles2Build
      mask Help: web('help_GPIOI_Config.html', '-helpbrowser')
      mask Callback Pin0_Use: GPIOI_Config_callback('use0');
      mask Callback Pin1_Use: GPIOI_Config_callback('use1');
      mask Callback Pin2_Use: GPIOI_Config_callback('use2');
      mask Callback Pin3_Use: GPIOI_Config_callback('use3');
      mask Callback Pin4_Use: GPIOI_Config_callback('use4');
      mask Callback Pin5_Use: GPIOI_Config_callback('use5');
      mask Callback Pin6_Use: GPIOI_Config_callback('use6');
      mask Callback Pin7_Use: GPIOI_Config_callback('use7');
      mask Callback Pin8_Use: GPIOI_Config_callback('use8');
      mask Callback Pin9_Use: GPIOI_Config_callback('use9');
      mask Callback Pin10_Use: GPIOA_Config_callback('use10');
      mask Callback Pin11_Use: GPIOI_Config_callback('use11');
      mask TypeOptions Pin0_Speed: GPIO_Speed_2MHz | GPIO_Speed_25MHz | GPIO_Speed_50MHz | GPIO_Speed_100MHz
      mask TypeOptions Pin1_Speed: GPIO_Speed_2MHz | GPIO_Speed_25MHz | GPIO_Speed_50MHz | GPIO_Speed_100MHz
      mask TypeOptions Pin2_Speed: GPIO_Speed_2MHz | GPIO_Speed_25MHz | GPIO_Speed_50MHz | GPIO_Speed_100MHz
      mask TypeOptions Pin3_Speed: GPIO_Speed_2MHz | GPIO_Speed_25MHz | GPIO_Speed_50MHz | GPIO_Speed_100MHz
      mask TypeOptions Pin4_Speed: GPIO_Speed_2MHz | GPIO_Speed_25MHz | GPIO_Speed_50MHz | GPIO_Speed_100MHz
      mask TypeOptions Pin5_Speed: GPIO_Speed_2MHz | GPIO_Speed_25MHz | GPIO_Speed_50MHz | GPIO_Speed_100MHz
      mask TypeOptions Pin6_Speed: GPIO_Speed_2MHz | GPIO_Speed_25MHz | GPIO_Speed_50MHz | GPIO_Speed_100MHz
      mask TypeOptions Pin7_Speed: GPIO_Speed_2MHz | GPIO_Speed_25MHz | GPIO_Speed_50MHz | GPIO_Speed_100MHz
      mask TypeOptions Pin8_Speed: GPIO_Speed_2MHz | GPIO_Speed_25MHz | GPIO_Speed_50MHz | GPIO_Speed_100MHz
      mask TypeOptions Pin9_Speed: GPIO_Speed_2MHz | GPIO_Speed_25MHz | GPIO_Speed_50MHz | GPIO_Speed_100MHz
      mask TypeOptions Pin10_Speed: GPIO_Speed_2MHz | GPIO_Speed_25MHz | GPIO_Speed_50MHz | GPIO_Speed_100MHz
      mask TypeOptions Pin11_Speed: GPIO_Speed_2MHz | GPIO_Speed_25MHz | GPIO_Speed_50MHz | GPIO_Speed_100MHz
      mask TypeOptions Pin0_Mode: GPIO_Mode_IN | GPIO_Mode_OUT | GPIO_Mode_AF | GPIO_Mode_AN
      mask Callback Pin0_Mode: GPIOI_Config_callback('mode0');
      mask TypeOptions Pin1_Mode: GPIO_Mode_IN | GPIO_Mode_OUT | GPIO_Mode_AF | GPIO_Mode_AN
      mask Callback Pin1_Mode: GPIOI_Config_callback('mode1');
      mask TypeOptions Pin2_Mode: GPIO_Mode_IN | GPIO_Mode_OUT | GPIO_Mode_AF | GPIO_Mode_AN
      mask Callback Pin2_Mode: GPIOI_Config_callback('mode2');
      mask TypeOptions Pin3_Mode: GPIO_Mode_IN | GPIO_Mode_OUT | GPIO_Mode_AF | GPIO_Mode_AN
      mask Callback Pin3_Mode: GPIOI_Config_callback('mode3');
      mask TypeOptions Pin4_Mode: GPIO_Mode_IN | GPIO_Mode_OUT | GPIO_Mode_AF | GPIO_Mode_AN
      mask Callback Pin4_Mode: GPIOA_Config_callback('mode4');
      mask TypeOptions Pin5_Mode: GPIO_Mode_IN | GPIO_Mode_OUT | GPIO_Mode_AF | GPIO_Mode_AN
      mask Callback Pin5_Mode: GPIOI_Config_callback('mode5');
      mask TypeOptions Pin6_Mode: GPIO_Mode_IN | GPIO_Mode_OUT | GPIO_Mode_AF | GPIO_Mode_AN
      mask Callback Pin6_Mode: GPIOI_Config_callback('mode6');
      mask TypeOptions Pin7_Mode: GPIO_Mode_IN | GPIO_Mode_OUT | GPIO_Mode_AF | GPIO_Mode_AN
      mask Callback Pin7_Mode: GPIOI_Config_callback('mode7');
      mask TypeOptions Pin8_Mode: GPIO_Mode_IN | GPIO_Mode_OUT | GPIO_Mode_AN
      mask Callback Pin8_Mode: GPIOI_Config_callback('mode8');
      mask TypeOptions Pin9_Mode: GPIO_Mode_IN | GPIO_Mode_OUT | GPIO_Mode_AF | GPIO_Mode_AN
      mask Callback Pin9_Mode: GPIOI_Config_callback('mode9');
      mask TypeOptions Pin10_Mode: GPIO_Mode_IN | GPIO_Mode_OUT | GPIO_Mode_AF | GPIO_Mode_AN
      mask Callback Pin10_Mode: GPIOI_Config_callback('mode10');
      mask TypeOptions Pin11_Mode: GPIO_Mode_IN | GPIO_Mode_OUT | GPIO_Mode_AF | GPIO_Mode_AN
      mask Callback Pin11_Mode: GPIOI_Config_callback('mode11');
      mask TypeOptions Pin0_Type: GPIO_OType_PP | GPIO_OType_OD
      mask TypeOptions Pin1_Type: GPIO_OType_PP | GPIO_OType_OD
      mask TypeOptions Pin2_Type: GPIO_OType_PP | GPIO_OType_OD
      mask TypeOptions Pin3_Type: GPIO_OType_PP | GPIO_OType_OD
      mask TypeOptions Pin4_Type: GPIO_OType_PP | GPIO_OType_OD
      mask TypeOptions Pin5_Type: GPIO_OType_PP | GPIO_OType_OD
      mask TypeOptions Pin6_Type: GPIO_OType_PP | GPIO_OType_OD
      mask TypeOptions Pin7_Type: GPIO_OType_PP | GPIO_OType_OD
      mask TypeOptions Pin8_Type: GPIO_OType_PP | GPIO_OType_OD
      mask TypeOptions Pin9_Type: GPIO_OType_PP | GPIO_OType_OD
      mask TypeOptions Pin10_Type: GPIO_OType_PP | GPIO_OType_OD
      mask TypeOptions Pin11_Type: GPIO_OType_PP | GPIO_OType_OD
      mask TypeOptions Pin0_PuPd: GPIO_PuPd_NOPULL | GPIO_PuPd_UP | GPIO_PuPd_DOWN
      mask TypeOptions Pin1_PuPd: GPIO_PuPd_NOPULL | GPIO_PuPd_UP | GPIO_PuPd_DOWN
      mask TypeOptions Pin2_PuPd: GPIO_PuPd_NOPULL | GPIO_PuPd_UP | GPIO_PuPd_DOWN
      mask TypeOptions Pin3_PuPd: GPIO_PuPd_NOPULL | GPIO_PuPd_UP | GPIO_PuPd_DOWN
      mask TypeOptions Pin4_PuPd: GPIO_PuPd_NOPULL | GPIO_PuPd_UP | GPIO_PuPd_DOWN
      mask TypeOptions Pin5_PuPd: GPIO_PuPd_NOPULL | GPIO_PuPd_UP | GPIO_PuPd_DOWN
      mask TypeOptions Pin6_PuPd: GPIO_PuPd_NOPULL | GPIO_PuPd_UP | GPIO_PuPd_DOWN
      mask TypeOptions Pin7_PuPd: GPIO_PuPd_NOPULL | GPIO_PuPd_UP | GPIO_PuPd_DOWN
      mask TypeOptions Pin8_PuPd: GPIO_PuPd_NOPULL | GPIO_PuPd_UP | GPIO_PuPd_DOWN
      mask TypeOptions Pin9_PuPd: GPIO_PuPd_NOPULL | GPIO_PuPd_UP | GPIO_PuPd_DOWN
      mask TypeOptions Pin10_PuPd: GPIO_PuPd_NOPULL | GPIO_PuPd_UP | GPIO_PuPd_DOWN
      mask TypeOptions Pin11_PuPd: GPIO_PuPd_NOPULL | GPIO_PuPd_UP | GPIO_PuPd_DOWN
      mask TypeOptions Pin0_AF: GPIO_AF_TIM5 | GPIO_AF_SPI2 | GPIO_AF_EVENTOUT
      mask TypeOptions Pin1_AF: GPIO_AF_SPI2 | GPIO_AF_DCMI | GPIO_AF_EVENTOUT
      mask TypeOptions Pin2_AF: GPIO_AF_TIM8 | GPIO_AF_SPI2 | GPIO_AF_I2S3ext | GPIO_AF_DCMI | GPIO_AF_EVENTOUT
      mask TypeOptions Pin3_AF: GPIO_AF_TIM8 | GPIO_AF_SPI2 | GPIO_AF_DCMI | GPIO_AF_EVENTOUT
      mask TypeOptions Pin4_AF: GPIO_AF_TIM8 | GPIO_AF_DCMI | GPIO_AF_EVENTOUT
      mask TypeOptions Pin5_AF: GPIO_AF_TIM8 | GPIO_AF_DCMI | GPIO_AF_EVENTOUT
      mask TypeOptions Pin6_AF: GPIO_AF_TIM8 | GPIO_AF_DCMI | GPIO_AF_EVENTOUT
      mask TypeOptions Pin7_AF: GPIO_AF_TIM8 | GPIO_AF_DCMI | GPIO_AF_EVENTOUT
      mask TypeOptions Pin9_AF: GPIO_AF_CAN1 | GPIO_AF_EVENTOUT
      mask TypeOptions Pin10_AF: GPIO_AF_ETH | GPIO_AF_EVENTOUT
      mask TypeOptions Pin11_AF: GPIO_AF_OTG_HS | GPIO_AF_EVENTOUT
      mask Display:
      | color('blue'); text(0.6, 0.90, 'STM32F4xx', 'horizontalalignment', 'right');color('black'); text(0.50, 0.12, 'GPIOI_Config', 'horizontalAlignment','center');
      | image(imread('ST.bmp','bmp'),'top-right');
  GPIO_Read : S-Function  FunctionName=GPIO_Read  Parameters=Port_name,Enable_sim  EnableBusSupport=off  mask(GPIO_Read){Port_name=GPIOA, Enable_sim=off}
      mask prompts: Port_name "Port Name"; Enable_sim "Enable simulation input:"
      mask help:
      | GPIO (General Purpose In/Out) Port read:
      | Read GPIOx 16bit value of port (A to I)
      mask Help: web('help_GPIO_Read.html', '-helpbrowser')
      mask TypeOptions Port_name: GPIOA | GPIOB | GPIOC | GPIOD | GPIOE | GPIOF | GPIOG | GPIOH | GPIOI
      mask Display:
      | color('blue'); text(0.6, 0.90, 'STM32F4xx', 'horizontalalignment', 'right');color('black'); text(0.50, 0.12, 'GPIO_Read', 'horizontalAlignment','center');
      | image(imread('ST.bmp','bmp'),'top-right');
      | port_label('output',1,'Out');
  GPIO_Write : S-Function  FunctionName=GPIO_Write  Parameters=Port_name,Enable_input,Pin0,Toggle_Pin0,Pin1,Toggle_Pin1,Pin2,Toggle_Pin2,Pin3,Toggle_Pin3,Pin4,Toggle_Pin4,Pin5,Toggle_Pin5,Pin6,Toggle_Pin6,Pin7,Toggle_Pin7,Pin8,Toggle_Pin8,Pin9,Toggle_Pin9,Pin10,Toggle_Pin10,Pin11,Toggle_Pin11,Pin12,Toggle_Pin12,Pin13,Toggle_Pin13,Pin14,Toggle_Pin14,Pin15,Toggle_Pin15  EnableBusSupport=off  mask(GPIO_Write){Port_name=GPIOA, Enable_input=off, Pin0=off, Toggle_Pin0=off, Pin1=off, Toggle_Pin1=off, Pin2=off, Toggle_Pin2=off, Pin3=off, Toggle_Pin3=off, Pin4=off, Toggle_Pin4=off, Pin5=off, Toggle_Pin5=off, Pin6=off, Toggle_Pin6=off, Pin7=off, Toggle_Pin7=off, Pin8=off, Toggle_Pin8=off, Pin9=off, Toggle_Pin9=off, Pin10=off, Toggle_Pin10=off, Pin11=off, Toggle_Pin11=off, Pin12=off, Toggle_Pin12=off, Pin13=off, Toggle_Pin13=off, Pin14=off, Toggle_Pin14=off, Pin15=off, Toggle_Pin15=off}
      mask prompts: Port_name "Port Name"; Enable_input "Enable input:"; Toggle_Pin0 "Toggle Pin0"; Toggle_Pin1 "Toggle Pin1"; Toggle_Pin2 "Toggle Pin2"; Toggle_Pin3 "Toggle Pin3"; Toggle_Pin4 "Toggle Pin4"; Toggle_Pin5 "Toggle Pin5"; Toggle_Pin6 "Toggle Pin6"; Toggle_Pin7 "Toggle Pin7"; Toggle_Pin8 "Toggle Pin8"; Toggle_Pin9 "Toggle Pin9"; Toggle_Pin10 "Toggle Pin10"; Toggle_Pin11 "Toggle Pin11"; Toggle_Pin12 "Toggle Pin12"; Toggle_Pin13 "Toggle Pin13"; Toggle_Pin14 "Toggle Pin14"; Toggle_Pin15 "Toggle Pin15"
      mask help:
      | GPIO (General Purpose In/Out) Port write:
      | Write GPIOx input value to selected pin(s) of port (A to I)
      | Only toggle is available when Enable input parameter is not set.
      mask init:
      | GPIO_Write_callback('init');
      mask Help: web('help_GPIO_Write.html', '-helpbrowser')
      mask TypeOptions Port_name: GPIOA | GPIOB | GPIOC | GPIOD | GPIOE | GPIOF | GPIOG | GPIOH | GPIOI
      mask Callback Enable_input: GPIO_Write_callback('Enable_input');
      mask Callback Pin0: GPIO_Write_callback('Pin0');
      mask Callback Toggle_Pin0: GPIO_Write_callback('Toggle0');
      mask Callback Pin1: GPIO_Write_callback('Pin1');
      mask Callback Toggle_Pin1: GPIO_Write_callback('Toggle1');
      mask Callback Pin2: GPIO_Write_callback('Pin2');
      mask Callback Toggle_Pin2: GPIO_Write_callback('Toggle2');
      mask Callback Pin3: GPIO_Write_callback('Pin3');
      mask Callback Toggle_Pin3: GPIO_Write_callback('Toggle3');
      mask Callback Pin4: GPIO_Write_callback('Pin4');
      mask Callback Toggle_Pin4: GPIO_Write_callback('Toggle4');
      mask Callback Pin5: GPIO_Write_callback('Pin5');
      mask Callback Toggle_Pin5: GPIO_Write_callback('Toggle5');
      mask Callback Pin6: GPIO_Write_callback('Pin6');
      mask Callback Toggle_Pin6: GPIO_Write_callback('Toggle6');
      mask Callback Pin7: GPIO_Write_callback('Pin7');
      mask Callback Toggle_Pin7: GPIO_Write_callback('Toggle7');
      mask Callback Pin8: GPIO_Write_callback('Pin8');
      mask Callback Toggle_Pin8: GPIO_Write_callback('Toggle8');
      mask Callback Pin9: GPIO_Write_callback('Pin9');
      mask Callback Toggle_Pin9: GPIO_Write_callback('Toggle9');
      mask Callback Pin10: GPIO_Write_callback('Pin10');
      mask Callback Toggle_Pin10: GPIO_Write_callback('Toggle10');
      mask Callback Pin11: GPIO_Write_callback('Pin11');
      mask Callback Toggle_Pin11: GPIO_Write_callback('Toggle11');
      mask Callback Pin12: GPIO_Write_callback('Pin12');
      mask Callback Toggle_Pin12: GPIO_Write_callback('Toggle12');
      mask Callback Pin13: GPIO_Write_callback('Pin13');
      mask Callback Toggle_Pin13: GPIO_Write_callback('Toggle13');
      mask Callback Pin14: GPIO_Write_callback('Pin14');
      mask Callback Toggle_Pin14: GPIO_Write_callback('Toggle14');
      mask Callback Pin15: GPIO_Write_callback('Pin15');
      mask Callback Toggle_Pin15: GPIO_Write_callback('Toggle15');
      mask Display:
      | color('blue'); text(0.6, 0.90, 'STM32F4xx', 'horizontalalignment', 'right');color('black'); text(0.50, 0.12, 'GPIO_Write', 'horizontalAlignment','center');
      | image(imread('ST.bmp','bmp'),'top-right');
      | input = get_param(gcbh,'Enable_input');
      | if isequal(input,'on')
      | port_label('input',1,'In');
      | end
